simulink model "EX66a"  (R2016b)
settings: Solver=ode3  StartTime=0.0  StopTime=10.005  FixedStep=2e-5  RelTol=1e-3  EnableMultiTasking=on
libraries: commfilt2 x1, commchan3 x1, commsink2 x1, commrandsrc2 x1
settings Model: Creator=Dennis Silage  LastModifiedBy=Silage
settings DataIOCC: LimitDataPoints=on  SaveFormat=Array  SignalLoggingSaveFormat=ModelDataLogs
settings OptimizationCC: ExpressionDepthLimit=2147483647  InitFltsAndDblsToZero=on  LifeSpan=inf
settings DebuggingCC: UnderspecifiedInitializationDetection=Classic  MergeDetectMultiDrivingBlocksExec=none  SolverPrmCheckMsg=warning  FcnCallInpInsideContextMsg=warning  StateNameClashWarn=warning  SFUnexpectedBacktrackingDiag=warning  SFNoUnconditionalDefaultTransitionDiag=warning  SFExecutionAtInitializationDiag=none
settings HardwareCC: ProdBitPerPointer=32  ProdBitPerSizeT=32  ProdBitPerPtrDiffT=32  ProdLargestAtomicFloat=None  ProdIntDivRoundTo=Undefined  ProdEndianess=Unspecified  ProdWordSize=32  ProdHWDeviceType=32-bit Generic
settings ModelReferenceCC: PropagateSignalLabelsOutOfModel=off
settings GRTTargetCC: TargetLangStandard=C89/C90 (ANSI)  GeneratePreprocessorConditionals=Disable all  CombineOutputUpdateFcns=off  GRTInterface=on
settings ConfigComp: CovMetricSettings=dw  CovHtmlReporting=on  CovSaveCumulativeToWorkspaceVar=on  CovSaveSingleToWorkspaceVar=on  CovExternalEMLEnable=off

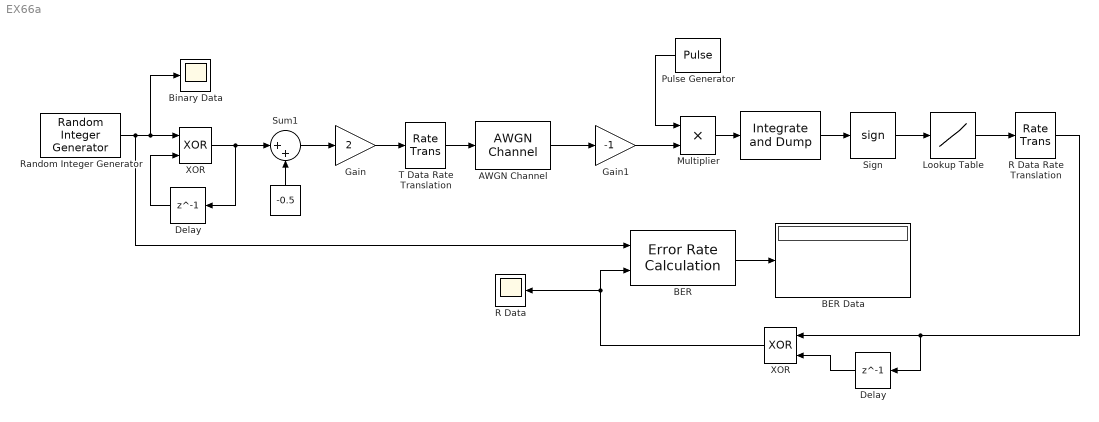
== system EX66a ==
  " " : commfilt2/Integrate and Dump  obssamples=50  offsetsamples=0  nodump=off  roundingMode=Floor  overflowMode=off
  "   " : Constant  Value=-0.5
  AWGN Channel : commchan3/AWGN Channel  InputProcessing=Inherited (this choice will be removed - see release notes)  seed=randseed  noiseMode=Variance from mask  EbNodB=90  EsNodB=10  SNRdB=10  bitsPerSym=1  Ps=25  Tsym=1e-3  variance=1
  BER : commsink2/Error Rate Calculation  N=2  st_delay=4  cp_mode=Entire frame  subframe=[]  PMode=Port  WsName=ErrorVec  RsMode2=off  stop=off  numErr=100  maxBits=1e6
  BER Data : Display
  Binary Data : Scope
  Delay : Delay  DelayLength=1  InitialCondition=0  UseCircularBuffer=on
  "Delay " : Delay  DelayLength=1  InitialCondition=0  InputProcessing=Columns as channels (frame based)
  Gain : Gain  Gain=2
  Gain1 : Gain  Gain=-1
  Lookup Table : Lookup  InputValues=[-1,0,1]  Table=[0,0,1]
  Multiplier : Product  RndMeth=Zero
  Pulse Generator : DiscretePulseGenerator  PulseType=Time based  Period=1e-3  PulseWidth=98
  R Data : Scope
  R Data Rate Translation : RateTransition  OutPortSampleTime=1e-3
  Random Integer Generator : commrandsrc2/Random Integer Generator  mul=2  seed=randseed  Ts=1e-3  frameBased=off  sampPerFrame=1  orient=off  outDataType=boolean
  Sign : Signum
  Sum1 : Sum  Inputs=|++
  "T Data Rate Translation  " : RateTransition
  XOR : Logic  Operator=XOR  IconShape=distinctive  AllPortsSameDT=off  OutDataTypeStr=boolean
  "XOR " : Logic  Operator=XOR  IconShape=distinctive  AllPortsSameDT=off  OutDataTypeStr=boolean
  wires:
  Random Integer Generator/1 -> XOR/1, Binary Data/1, BER/1
  "   "/1 -> Sum1/2
  Sum1/1 -> Gain/1
  Gain/1 -> "T Data Rate Translation  "/1
  XOR/1 -> Delay/1, Sum1/1
  Delay/1 -> XOR/2
  BER/1 -> BER Data/1
  Multiplier/1 -> " "/1
  " "/1 -> Sign/1
  Pulse Generator/1 -> Multiplier/1
  "T Data Rate Translation  "/1 -> AWGN Channel/1
  Sign/1 -> Lookup Table/1
  "Delay "/1 -> "XOR "/2
  Lookup Table/1 -> R Data Rate Translation/1
  R Data Rate Translation/1 -> "XOR "/1, "Delay "/1
  "XOR "/1 -> BER/2, R Data/1
  AWGN Channel/1 -> Gain1/1
  Gain1/1 -> Multiplier/2
